simulink model "Test_gmt_Simulink"  (R2025a)
settings: Solver=ode23s  StartTime=0.0  StopTime=1000  MinStep=eps  RelTol=1e-3
undefined symbols (not defined in the file or in its folder): TT, y0
libraries: slpidlib x1
settings Model: Creator=jmp8430  LastModifiedBy=jmp8430

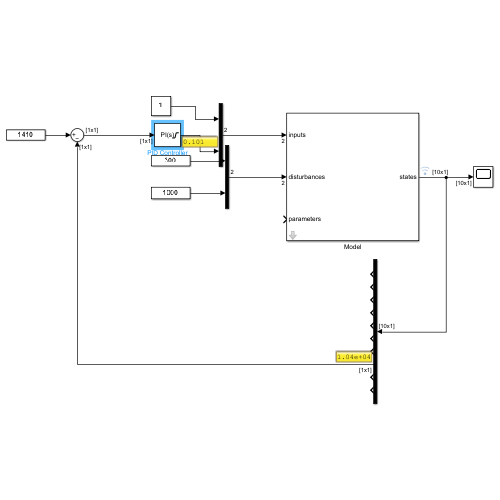
[thumbnail: Simulink's stored preview of the top-level diagram]
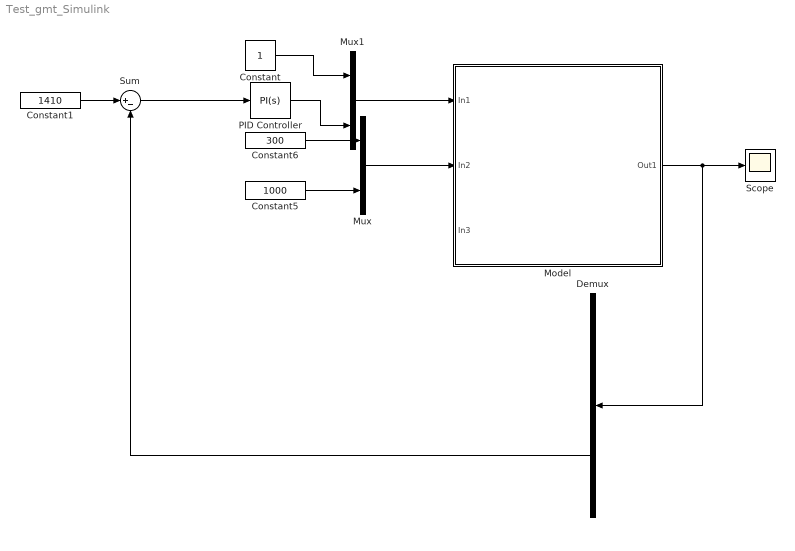
== system Test_gmt_Simulink ==
  Constant : Constant
  Constant1 : Constant  Value=1410
  Constant5 : Constant  Value=1000
  Constant6 : Constant  Value=300
  Demux : Demux  Outputs=10
  Model : Subsystem  mask{mdlName=TT, x0=y0', x0_workspace_flg=on}
      mask prompts: mdlName "Model Name (must be object in working directory)"; x0 "Initial State (10):"; x0_workspace_flg "Pull initial conditions from workspace object?"
      settings: CopyFcn=set_param(gcb, 'LinkStatus', 'none');
      mask Callback mdlName:
      | try
      |         blkPath = gcb;
      |         maskObj = Simulink.Mask.get(blkPath);
      |         maskWorkspace = maskObj.getWorkspace();
      |         parameterObj = maskObj.getParameter('mdlName');
      | 
      |         disp('mdlName update callback triggered');
      |         graphObj_name = parameterObj.Value;
      | 
      |         %% Verify variable is in MATLAB workspace (base)
      |         inMATLABworkspace = evalin('base', ['exist(''', graphObj_name, ''', ''var'')']);
      |         assert(inMATLABworkspace,"Variable selected not in MATLAB workspace")
      | 
      |         %% Create graph object variable and verify object is gmt_Graph class
      |         graphObj = evalin('base', graphObj_name);
      |         isGraphObj = isa(graphObj,"gmt_Graph");
      |         assert(isGraphObj,"Variable selected is not a gmt_Graph class")
      | 
      |         %% Grab Basic Graph Object Properties
      |         Nx = graphObj.Properties.Ns;
      |         Ny = graphObj.Properties.Ny;
      |         Nd = graphObj.Properties.Nd;
      |         Nu = graphObj.Properties.Nu;
      |         opt_idx = [graphObj.ModelParameters.Optimization] == true;
      |         Nopt = sum(opt_idx);
      | 
      |         %% Create Mask Prompts
      |         State_Prompt = vertcat(graphObj.States' + ": " + [graphObj.Vertices(graphObj.Properties.Ns_idx).VertexName]');
      |         Output_Prompt = vertcat(graphObj.Outputs);
      |         Input_Prompt = vertcat(graphObj.Inputs' + ": " + [graphObj.InputData.Parent]' + " " + [graphObj.InputData.Description]');
      |         Disturbance_Prompt = vertcat(graphObj.Disturbances' + ": " + [graphObj.Vertices(graphObj.Properties.Nd_idx).VertexName]');
      |         Parameter_Prompt = vertcat([graphObj.ModelParameters(opt_idx).Variable]'+ ": " + [graphObj.ModelParameters(opt_idx).Description]');
      |         CurrentModel_Prompt = "Current Model Loaded: " + parameterObj.Value;
      |         InitialCondition_Prompt = "Initial State (" + string(Nx) + "):";
      | 
      |         %% Update States Info
      |         tbObj = maskObj.getDialogControl("States");
      |         prompt_tmp = State_Prompt;
      | 
      |         if ~isempty(prompt_tmp)
      |             if length(prompt_tmp) > 1
      |                 % set the Prompt value
      |                 tbObj.Prompt = strjoin(convertStringsToChars(prompt_tmp),newline);
      |             else
      |                 tbObj.Prompt = prompt_tmp;
      |             end
      |         else
      |             % set the Prompt value
      |             tbObj.Prompt = "";
      |         end
      | 
      |         %% Update Inputs Info
      |         tbObj = maskObj.getDialogControl("Inputs");
      |         prompt_tmp = Input_Prompt;
      | 
      |         if ~isempty(prompt_tmp)
      |             if length(prompt_tmp) > 1
      |                 % set the Prompt value
      |                 tbObj.Prompt = strjoin(convertStringsToChars(prompt_tmp),newline);
      |             else
      |                 tbObj.Prompt = prompt_tmp;
      |             end
      |         else
      |             % set the Prompt value
      |             tbObj.Prompt = "";
      |         end
      | 
      |         %% Update Outputs Info
      |         tbObj = maskObj.getDialogControl("Outputs");
      |         prompt_tmp = Output_Prompt;
      | 
      |         if ~isempty(prompt_tmp)
      |             if length(prompt_tmp) > 1
      |                 % set the Prompt value
      |                 tbObj.Prompt = strjoin(convertStringsToChars(prompt_tmp),newline);
      |             else
      |                 tbObj.Prompt = prompt_tmp;
      |             end
      |         else
      |             % set the Prompt value
      |             tbObj.Prompt = "";
      |         end
      | 
      |         %% Update Parameters Info
      |         tbObj = maskObj.getDialogControl("Parameters");
      |         prompt_tmp = Parameter_Prompt;
      | 
      |         if ~isempty(prompt_tmp)
      |             if length(prompt_tmp) > 1
      |                 % set the Prompt value
      |                 tbObj.Prompt = strjoin(convertStringsToChars(prompt_tmp),newline);
      |             else
      |                 tbObj.Prompt = prompt_tmp;
      |             end
      |         else
      |             % set the Prompt value
      |             tbObj.Prompt = "";
      |         end
      | 
      |         %% Update Disturbances Info
      |         tbObj = maskObj.getDialogControl("Disturbances");
      |         prompt_tmp = Disturbance_Prompt;
      | 
      |         if ~isempty(prompt_tmp)
      |             if length(prompt_tmp) > 1
      |                 % set the Prompt value
      |                 tbObj.Prompt = strjoin(convertStringsToChars(prompt_tmp),newline);
      |             else
      |                 tbObj.Prompt = prompt_tmp;
      |             end
      |         else
      |             % set the Prompt value
      |             tbObj.Prompt = "";
      |         end
      | 
      |         %% Update mdlName_current Info
      |         tbObj = maskObj.getDialogControl("mdlName_current");
      |         prompt_tmp = CurrentModel_Prompt;
      | 
      |         if ~isempty(prompt_tmp)
      |             if length(prompt_tmp) > 1
      |                 % set the Prompt value
      |                 tbObj.Prompt = strjoin(convertStringsToChars(prompt_tmp),newline);
      |             else
      |                 tbObj.Prompt = prompt_tmp;
      |             end
      |         else
      |             % set the Prompt value
      |             tbObj.Prompt = "";
      |         end
      | 
      |         %% Update Initial Condition Number
      |         tbObj = maskObj.getParameter('x0');
      |         tbObj.Prompt = "Initial State (" + string(Nx) + "):";
      | 
      |         %% Add Initial Conditions
      |         paramObj = maskObj.getParameter('x0_workspace_flg');
      |         rawValue = paramObj.Value;
      |         if strcmp(string(rawValue),"on")
      |             tbObj = maskObj.getParameter('x0');
      |             initCon_values = graphObj.InitialConditions;
      |             %assert(initCon_values,"No initial conditions specified in model")
      |             initCon_str = "[" + strjoin(string(initCon_values),";") + "]";
      |             tbObj.Value = initCon_str;
      |         end
      | 
      |         disp("Updated mask with model info")
      | 
      |          %% Update MATLAB Function Code
      |         blkPath = gcb;
      |         rt = sfroot;
      |         funcBlk = rt.find('-isa', 'Stateflow.EMChart', '-and', 'Path', [blkPath '/MATLAB Function']);
      | 
      |         %% MATLAB Function Prefix
      | 
      |         % Grab State Variable Names
      |         StateVars = graphObj.States';
      |         % Grab Boundary Condition Variable Names
      |         ExtAlgVars = graphObj.Disturbances';
      |         % Grab Control Input Variable Names
      |         InputVars = graphObj.Inputs';
      |         % System Input Packager
      |         funcInput_list = [StateVars; InputVars; ExtAlgVars];
      |         sysfun_mfile_prefix = "";
      |         for i = 1:length(funcInput_list)
      |             sysfun_mfile_prefix(i,1) = funcInput_list(i) + " = u(" + i + ");";
      |         end
      |         %% MATLAB Function Parameters
      |         sysfun_mfile_param = graphObj.ModelMetadata.mfileCode_param;
      |         %% MATLAB Function Body
      |         stateVars_der = StateVars + "_dot";
      |         sysfun_mfile_body = stateVars_der + " = " +  string(graphObj.SystemEquations.RHS) + ";";
      |         %% MATLAB Function Suffix
      |         sysfun_mfile_suffix = "y = [" + strjoin(stateVars_der',";") + "];";
      |         sysfun_mfile_suffix = [sysfun_mfile_suffix; "end"];
      |         %% Create newCode
      |         newCode_str = [sysfun_mfile_prefix;sysfun_mfile_param;sysfun_mfile_body;sysfun_mfile_suffix];
      |         newCode = strjoin(newCode_str,'\n');
      |         funcBlk.Script = newCode;
      | 
      |         %% Update Port Dimensions
      |         totInputs = Nx + Nd + Nu + Nopt;
      |         totOutputs = Nx;
      | 
      |         disp(string(totOutputs))
      |         funcBlk.Inputs.Props.Array.isDynamic = true;
      |         funcBlk.Inputs.Props.Array.Size = "[" + string(totInputs) + " " + string(1) + "]";
      |         funcBlk.Outputs.Props.Array.isDynamic = true;
      |         if totOutputs > 1
      |             funcBlk.Outputs.Props.Array.Size = "[" + string(totOutputs) + " " + string(1) + "]";
      |         else
      |             funcBlk.Outputs.Props.Array.Size =  string(1);
      |         end
      |             disp(funcBlk.Inputs.Props.Array)
      |         disp(funcBlk.Outputs.Props.Array)
      | 
      |         %% Update Mux Dimensions
      |         muxPath = [blkPath '/Mux'];
      |         muxHdl  = get_param(muxPath, 'Handle');
      |         muxPortHdl = get_param(muxPath, 'PortHandles');
      | 
      | 
      |         % Break All Input Lines Into Mux
      |         for k = 1:length(muxPortHdl.Inport)
      |         line = get_param(muxPortHdl.Inport(k), 'Line');
      |             if line ~= -1   % -1 means no line connected
      |                 delete_line(line);
      |             end
      |         end
      | 
      |         % Find and Delete all Terminators
      |         %terms = find_system(blkPath, 'BlockType', 'Terminator', 'LookUnderMasks','all', 'FollowLinks','on');
      | 
      |         %for k = 1:length(terms)
      |         %    delete_block(terms{k});
      |         %end
      | 
      |         % Compute Mux Dimensions
      |         muxNum = 1;
      |         if Nd > 0
      |             muxNum = muxNum + 1;
      |         end
      | 
      |         if Nu > 0
      |             muxNum = muxNum + 1;
      |         end
      | 
      |         if Nopt > 0
      |             muxNum = muxNum + 1;
      |         end
      | 
      |         set_param(muxHdl, 'Inputs', string(muxNum));   % set to 3 inputs
      | 
      |         % Connect Integrator
      |         integratorPath = [blkPath '/Integrator'];
      |         integratorHdl  = get_param(integratorPath, 'Handle');
      |         integratorPortHdl = get_param(integratorPath, 'PortHandles');
      |         add_line(blkPath, integratorPortHdl.Outport(1), muxPortHdl.Inport(1), 'autorouting','on');
      |         PortNum = 1;
      | 
      |         % Connect In1
      |         if Nu > 0
      |             PortNum = PortNum + 1;
      |             In1Path = [blkPath '/In1'];
      |             In1Hdl  = get_param(In1Path, 'Handle');
      |             In1PortHdl = get_param(In1Path, 'PortHandles');
      |             add_line(blkPath, In1PortHdl.Outport(1), muxPortHdl.Inport(PortNum), 'autorouting','on');
      |         else
      | 
      |         end
      | 
      |         % Connect In2
      |         if Nd > 0
      |             PortNum = PortNum + 1;
      |             In2Path = [blkPath '/In2'];
      |             In2Hdl  = get_param(In2Path, 'Handle');
      |             In2PortHdl = get_param(In2Path, 'PortHandles');
      |             add_line(blkPath, In2PortHdl.Outport(1), muxPortHdl.Inport(PortNum), 'autorouting','on');
      |         end
      | 
      |         % Connect In3
      |         if Nopt > 0
      |             PortNum = PortNum + 1;
      |             In3Path = [blkPath '/In3'];
      |             In3Hdl  = get_param(In3Path, 'Handle');
      |             In3PortHdl = get_param(In3Path, 'PortHandles');
      |             add_line(blkPath, In3PortHdl.Outport(1), muxPortHdl.Inport(PortNum), 'autorouting','on');
      |         end
      | 
      |     catch ME
      |         disp(getReport(ME, 'extended'))
      |         rethrow(ME)  % still show Simulink error dialog
      |     end
      mask DialogControl Container7 Prompt: Description
      mask DialogControl Control6 Prompt: This Simulink block can be used to load and simulate a model generated and saved with the graph modeling toolbox. The only input requirements are the model's workspace object name.
      mask DialogControl DescGroupVar Prompt: States
      mask DialogControl States Prompt:
      | x2: TT: Low Pressure Compressor - Temperature
      | x3: TT: High Pressure Compressor - Temperature
      | x4: TT: Combustion Chamber - Temperature
      | x5: TT: Fuel Tank - Temperature
      | x6: TT: High Pressure Turbine - Temperature
      | x7: TT: High Pressure Turbine - Angular Velocity
      | x8: TT: Low Pressure Turbine - Temperature
      | x9: TT: Low Pressure Turbine - Angular Velocity
      | x10: TT: Power Turbine - Temperature
      | x11: TT: Power Turbine - Angular Velocity
      mask DialogControl Container3 Prompt: Outputs
      mask DialogControl Container4 Prompt: Inputs
      mask DialogControl Inputs Prompt:
      | u1: TT Inlet Air Mass Flow
      | u2: TT Inlet Fuel Mass Flow
      mask DialogControl Container5 Prompt: Disturbances
      mask DialogControl Disturbances Prompt:
      | x1: TT: Source - Temperature
      | x13: TT: Sink - Mechanical
      mask DialogControl Container6 Prompt: Parameters
      mask DialogControl ParameterGroupVar Prompt: Model Configuration
      mask DialogControl mdlName_current Prompt: Current Model Loaded: TT
      mask Display:
      | port_label('input', 1, 'inputs');
      | port_label('input', 2, 'disturbances');
      | port_label('input', 3, 'parameters');
      | port_label('output', 1, 'states');
  Mux : Mux  Inputs=2
  Mux1 : Mux  Inputs=2
  PID Controller : slpidlib/PID Controller  Controller=PI  Form=Parallel  TimeDomain=Continuous-time  UseExternalTs=off  SampleTime=-1  IntegratorMethod=Forward Euler  FilterMethod=Forward Euler  ControllerParametersSource=internal  P=0.0001  I=0.00001  UseKiTs=off  D=0  UseExternalDerivativeSource=off  N=100  UseFilter=on  TunerSelectOption=Transfer Function Based (PID Tuner App)  InitialConditionSource=internal  InitialConditionForIntegrator=1  InitialConditionForFilter=0  DifferentiatorICPrevScaledInput=0  ExternalReset=none  TrackingMode=off  Kt=1  LimitOutput=on  SatLimitsSource=internal  UpperSaturationLimit=1  LowerSaturationLimit=0  LinearizeAsGain=on  AntiWindupMode=clamping  Kb=1  LimitIntegrator=off  UpperIntegratorSaturationLimit=inf  LowerIntegratorSaturationLimit=-inf  POutMin=[]  POutMax=[]  IOutMin=[]  IOutMax=[]  DOutMin=[]  DOutMax=[]  NOutMin=[]  NOutMax=[]  SumOutMin=[]  SumOutMax=[]  SaturationOutMin=[]  SaturationOutMax=[]  PParamMin=[]  PParamMax=[]  IParamMin=[]  IParamMax=[]  DParamMin=[]  DParamMax=[]  NParamMin=[]  NParamMax=[]  KbParamMin=[]  KbParamMax=[]  KtParamMin=[]  KtParamMax=[]  KbOutMin=[]  KbOutMax=[]  KtOutMin=[]  KtOutMax=[]  IntegratorOutMin=[]  IntegratorOutMax=[]  FilterOutMin=[]  FilterOutMax=[]  SumI1OutMin=[]  SumI1OutMax=[]  SumI2OutMin=[]  SumI2OutMax=[]  SumI3OutMin=[]  SumI3OutMax=[]  SumI4OutMin=[]  SumI4OutMax=[]  SumDOutMin=[]  SumDOutMax=[]  DifferentiatorOutMin=[]  DifferentiatorOutMax=[]  FilterDiffOutCoefMin=[]  FilterDiffOutCoefMax=[]  ReciprocalOutMin=[]  ReciprocalOutMax=[]  SumDenOutMin=[]  SumDenOutMax=[]  SumNumOutMin=[]  SumNumOutMax=[]  DivideOutMin=[]  DivideOutMax=[]  UdiffTsProdOutMin=[]  UdiffTsProdOutMax=[]  NTsProdOutMin=[]  NTsProdOutMax=[]  UintegralTsProdOutMin=[]  UintegralTsProdOutMax=[]  UngainTsProdOutMin=[]  UngainTsProdOutMax=[]  ClampingZeroOutDataTypeStr=Inherit: Inherit via back propagation  ClampingZeroOutMin=[]  ClampingZeroOutMax=[]  FilterDenConstantOutDataTypeStr=Inherit: Inherit via back propagation  FilterDenConstantOutMin=[]  FilterDenConstantOutMax=[]  PCopyOutDataTypeStr=Inherit: Inherit via back propagation  PCopyOutMin=[]  PCopyOutMax=[]  NCopyOutDataTypeStr=Inherit: Inherit via back propagation  NCopyOutMin=[]  NCopyOutMax=[]  IntegratorContinuousStateAttributes=''  IntegratorStateMustResolveToSignalObject=off  IntegratorRTWStateStorageClass=Auto  FilterContinuousStateAttributes=''  FilterStateMustResolveToSignalObject=off  FilterRTWStateStorageClass=Auto  ParallelPVariant=InternalParameters  IdealPVariant=Disabled  IVariant=InternalParameters  DVariant=Disabled  IntegratorVariant=Continuous  SatVariant=Enabled  AWVariant=ContClampingParallel  PCopyVariant=Disabled  TRVariant=Disabled  FdbkBlocksVariant=Forward  IdealPFdbkVariant=Disabled  SatFdbkVariant=Disabled  DerivativeFilterVariant=Disabled  NVariant=Disabled  NCopyVariant=Disabled_SignalSpec  FilterICVariant=Disabled  IntegratorICVariant=InternalICs  ExternalResetVariant=Disabled  TRSumVariant=Passthrough  SumFdbkVariant=Disabled  SumVariant=Sum_PI  TsampFilterVariant=InternalTs  TsampNgainVariant=Passthrough  TsampIntegralVariant=Disabled_SignalSpec  ExternalSaturationOutDataTypeStr=Inherit: Same as second input  DerivativeSourceVariant=Disabled  PreIntVariant=InternalPreInt
  Scope : Scope
      settings: ActiveDisplayYMinimum=-1  ActiveDisplayYMaximum=1
  Sum : Sum  Inputs=|+-
  wires:
  Mux/1 -> Model/2(In2)
  Model/1(Out1) -> Demux/1, Scope/1
  Constant6/1 -> Mux/1
  Constant5/1 -> Mux/2
  PID Controller/1 -> Mux1/2
  Sum/1 -> PID Controller/1
  Constant1/1 -> Sum/1
  Demux/8 -> Sum/2
  Mux1/1 -> Model/1(In1)
  Constant/1 -> Mux1/1

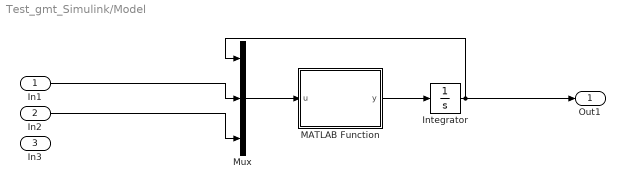
== system Test_gmt_Simulink/Model ==
  In1 : Inport
  In2 : Inport  Port=2
  In3 : Inport  Port=3
  Integrator : Integrator  InitialCondition=x0
  MATLAB Function : MATLAB Function  TreatAsAtomicUnit=on
  Mux : Mux  Inputs=3
  Out1 : Outport
  wires:
  MATLAB Function/1(y) -> Integrator/1
  Integrator/1 -> Out1/1, Mux/1
  Mux/1 -> MATLAB Function/1(u)
  In1/1 -> Mux/2
  In2/1 -> Mux/3

== matlab function Test_gmt_Simulink/Model/MATLAB Function ==
  data: u input size=[14 1]; y output size=[10 1]
function y = fcn(u)
x2 = u(1);
x3 = u(2);
x4 = u(3);
x5 = u(4);
x6 = u(5);
x7 = u(6);
x8 = u(7);
x9 = u(8);
x10 = u(9);
x11 = u(10);
u1 = u(11);
u2 = u(12);
x1 = u(13);
x13 = u(14);
cp_f = 1000;
Rho = 1.25;
V1 = 0.002;
V2 = 0.002;
V3 = 0.002;
V4 = 0.002;
V5 = 0.002;
V6 = 0.002;
LPJ = 0.1;
HPJ = 0.1;
PTJ = 0.1;
LHV = 43000000;
PTwref = 100;
HPT_p00 = 71.1041427121;
HPT_p10 = -0.453128884834;
HPT_p01 = 0.152865555398;
HPT_p11 = 0.000290828633908;
HPT_p02 = -6.77543050801e-05;
HPT_p12 = -2.82439223155e-08;
HPT_p03 = 6.73633771983e-09;
HPC_p00 = 791.959214833;
HPC_p10 = -2.11873391303;
HPC_p01 = -0.212071998241;
HPC_p11 = 0.00112820832044;
HPC_p02 = -1.87370155433e-05;
HPC_p12 = -1.09394503401e-07;
HPC_p03 = 5.23642741344e-09;
LPT_p00 = 197.216269388;
LPT_p10 = -0.262766227573;
LPT_p01 = 0.0262095014054;
LPT_p11 = 0.000215319839135;
LPT_p02 = -3.59106246598e-05;
LPT_p12 = -2.20942011219e-08;
LPT_p03 = 4.48379908676e-09;
LPC_p00 = 414.859315297;
LPC_p10 = -1.18070744809;
LPC_p01 = -0.12661181663;
LPC_p11 = 0.000769070197029;
LPC_p02 = -3.60584711554e-06;
LPC_p12 = -6.36957284105e-08;
LPC_p03 = 1.7282571386e-09;
PT_p1 = 9.31016581174e-07;
PT_p2 = 1.2505492566e-05;
PT_p3 = 0.337662266024;
PT_p4 = 31.5146029489;
x2_dot = (0.97*LPC_p00*x2 + 0.97*LPC_p01*x9^2 + 0.97*LPC_p02*x9^3 + 0.97*LPC_p03*x9^4 + 0.97*LPC_p10*x2*x9 + cp_f*u1*x1 - cp_f*u1*x2 + 0.97*LPC_p11*x2*x9^2 + 0.97*LPC_p12*x2*x9^3)/(Rho*V1*cp_f);
x3_dot = (0.97*HPC_p00*x7 + 0.97*HPC_p01*x7^2 + 0.97*HPC_p02*x7^3 + 0.97*HPC_p03*x7^4 + 0.97*HPC_p10*x3*x7 + cp_f*u1*x2 - cp_f*u1*x3 + 0.97*HPC_p11*x3*x7^2 + 0.97*HPC_p12*x3*x7^3)/(Rho*V2*cp_f);
x4_dot = (LHV*u2 + cp_f*u1*x3 - cp_f*u1*x4)/(Rho*V3*cp_f);
x5_dot = -(LHV*u2)/(Rho*V3*cp_f);
x6_dot = -(0.97*HPT_p00*x7 + 0.97*HPT_p01*x7^2 + 0.97*HPT_p02*x7^3 + 0.97*HPT_p03*x7^4 + 0.97*HPT_p10*x6*x7 - cp_f*u1*x4 + cp_f*u1*x6 + 0.97*HPT_p11*x6*x7^2 + 0.97*HPT_p12*x6*x7^3)/(Rho*V4*cp_f);
x7_dot = -(0.97*HPC_p00*x7 - 0.97*HPT_p00*x7 + 0.97*HPC_p01*x7^2 + 0.97*HPC_p02*x7^3 + 0.97*HPC_p03*x7^4 - 0.97*HPT_p01*x7^2 - 0.97*HPT_p02*x7^3 - 0.97*HPT_p03*x7^4 + 0.97*HPC_p10*x3*x7 - 0.97*HPT_p10*x6*x7 + 0.97*HPC_p11*x3*x7^2 + 0.97*HPC_p12*x3*x7^3 - 0.97*HPT_p11*x6*x7^2 - 0.97*HPT_p12*x6*x7^3)/(HPJ*x7);
x8_dot = -(0.97*LPT_p00*x9 + 0.97*LPT_p01*x9^2 + 0.97*LPT_p02*x9^3 + 0.97*LPT_p03*x9^4 + 0.97*LPT_p10*x8*x9 - cp_f*u1*x6 + cp_f*u1*x8 + 0.97*LPT_p11*x8*x9^2 + 0.97*LPT_p12*x8*x9^3)/(Rho*V5*cp_f);
x9_dot = -(0.97*LPC_p00*x2 - 0.97*LPT_p00*x9 + 0.97*LPC_p01*x9^2 + 0.97*LPC_p02*x9^3 + 0.97*LPC_p03*x9^4 - 0.97*LPT_p01*x9^2 - 0.97*LPT_p02*x9^3 - 0.97*LPT_p03*x9^4 + 0.97*LPC_p10*x2*x9 - 0.97*LPT_p10*x8*x9 + 0.97*LPC_p11*x2*x9^2 + 0.97*LPC_p12*x2*x9^3 - 0.97*LPT_p11*x8*x9^2 - 0.97*LPT_p12*x8*x9^3)/(LPJ*x9);
x10_dot = -(PT_p4*PTwref - PT_p4*x11 + PT_p3*PTwref*x10 - PT_p3*x10*x11 - cp_f*u1*x8 + cp_f*u1*x10 + PT_p1*PTwref*x10^3 + PT_p2*PTwref*x10^2 - PT_p1*x10^3*x11 - PT_p2*x10^2*x11)/(Rho*V6*cp_f);
x11_dot = -(PT_p4*x11 - PT_p4*PTwref + x11*x13 - PT_p3*PTwref*x10 + PT_p3*x10*x11 - PT_p1*PTwref*x10^3 - PT_p2*PTwref*x10^2 + PT_p1*x10^3*x11 + PT_p2*x10^2*x11)/(PTJ*x11);
y = [x2_dot;x3_dot;x4_dot;x5_dot;x6_dot;x7_dot;x8_dot;x9_dot;x10_dot;x11_dot];
end
